simulink model "DFADAS2_SenFus_v1_201204RC_training_210115"  (R2018b)
settings: Solver=FixedStepDiscrete  StartTime=0.0  StopTime=inf  FixedStep=0.002  RelTol=1e-3  EnableMultiTasking=on
PreLoadFcn:
  | RTWConfigurationCB('preloadfcn', bdroot);
libraries: canmsglib x108, simulink x48, canfdmsglib x12
(part 12 of 28)

== system DFADAS2_SenFus_v1_201204RC_training_210115/Signal Input (Input)/Signal Input (10ms) (Input10)/VehInfo/Vehicle Movement Signal Receive and Processing (VehMovRx)/Yaw State CAN Frame PreProcess (YawCANFrmPPrcs) ==
  CAN Diagnosis (CANDia) : Subsystem  Commented=on
  CAN Receive Sample Time : Constant  Value=0.02  OutDataTypeStr=single  SampleTime=-1
  CAN Unpack : canmsglib/CAN Unpack  CANdbFile=F:\LD\3_simulinkModel_13b\TJAHWA\ADAS_D53_PSA1CAN_LiPiao_DLC.dbc  MsgList=ESC_3CD_PSA1  MsgName=ESC_3CD_PSA1  MsgIDType=Standard (11-bit identifier)  MsgIdentifier=973  MsgLength=8  SignalInfo=Brake_pedal_disabled_UC_Brake$37$1$2$2$1$0$1$0$-Inf$Inf$#Frame_checksum3CD$60$4$2$2$1$0$1$0$-Inf$Inf$#Lateral_acceleration$8$16$2$1$1$0$5.000000e-02$0$-15$15$#TMC_pressure$52$12$2$2$1$0$1.000000e-01$-55$-55$3.544000e+02$#Yaw_speed$24$16$2$1$1$0$1.000000e-01$0$-100$100$#bits_compute_process_counter3CD$56$4$2$2$1$0$1$0$0$15$#  NSignals=6  IDPort=off  TimestampPort=off  ErrorPort=off  RemotePort=off  LengthPort=off  StatusPort=off  StartBits=str2num('[int32(37);int32(60);int32(8);int32(52);int32(24);int32(56)]')  SignalSizes=str2num('[int32(1);int32(4);int32(16);int32(12);int32(16);int32(4)]')  ByteOrders=str2num('[int32(2);int32(2);int32(2);int32(2);int32(2);int32(2)]')  DataTypes=str2num('[int32(2);int32(2);int32(1);int32(2);int32(1);int32(2)]')  MultiplexTypes=str2num('[int32(1);int32(1);int32(1);int32(1);int32(1);int32(1)]')  MultiplexValues=str2num('[double(0);double(0);double(0);double(0);double(0);double(0)]')  Factors=str2num('[double(1);double(1);double(5.000000e-02);double(1.000000e-01);double(1.000000e-01);double(1)]')  Offsets=str2num('[double(0);double(0);double(0);double(-55);double(0);double(0)]')  Minimums=str2num('[double(-Inf);double(-Inf);double(-15);double(-55);double(-100);double(0)]')  Maximums=str2num('[double(Inf);double(Inf);double(15);double(3.544000e+02);double(100);double(15)]')  ApplyMinMax=off
      settings: SourceProductName=Simulink Real-Time  SourceProductBaseCode=XP  DataFormat=CANdb specified signals
  Data Type Conversion{2..5} (4 alike) : DataTypeConversion  OutDataTypeStr=single
  Data Type Conversion55 : DataTypeConversion  OutDataTypeStr=uint16
  Rate Transition{1..5} (5 alike) : RateTransition  OutPortSampleTime=0.01
  S-Function1 : S-Function  FunctionName=NSTC297CANReceiveBlkLib  Parameters=|  SFunctionDeploymentMode=off  EnableBusSupport=off  mask(NSTC297 CAN Receive){Ns_DeviceID=ADAS Control Unit Gen2, Ns_ChannelNum=4, Ns_FrameID=973, Ns_IsVirtualFrame=off, Ns_RoleInVirtualFrame=Header Frame, Ns_HeaderFrameID=0, Ns_VirtualFrameStatusFlg=off, Ns_IncompleteFrameCntFlg=off, Ns_OverflowCntFlg=off, Ns_FrameBufferSize=1, Ns_SampleTime=0.01}
      | uint16(Ns_DeviceID),
      | uint16(Ns_ChannelNum),
      | uint32(Ns_FrameID),
      | uint8(Ns_IsVirtualFrame),
      | uint16(Ns_RoleInVirtualFrame),
      | uint32(Ns_HeaderFrameID),
      | uint8(Ns_VirtualFrameStatusFlg),
      | uint8(Ns_IncompleteFrameCntFlg),
      | uint8(Ns_OverflowCntFlg),
      | uint16(Ns_FrameBufferSize),
      | double(Ns_SampleTime)
      mask prompts: Ns_DeviceID "Device:"; Ns_ChannelNum "Channel number:"; Ns_FrameID "Frame ID:"; Ns_IsVirtualFrame "Belong to a virtual frame"; Ns_RoleInVirtualFrame "Position in virtual frame:"; Ns_HeaderFrameID "Header frame ID:"; Ns_VirtualFrameStatusFlg "Current virtural frame status output"; Ns_IncompleteFrameCntFlg "Incomplete virtual frame count output"; Ns_OverflowCntFlg "Overflow count output"; Ns_FrameBufferSize "Frame buffer size:"; Ns_SampleTime "Sample time:"
      mask init:
      | NSTC297CANReceive_callback('portlabels');
      mask TypeOptions Ns_DeviceID: General Control Unit Gen2 | ADAS Control Unit Gen2
      mask TypeOptions Ns_ChannelNum: 0 | 1 | 2 | 3 | 4 | 5
      mask Callback Ns_IsVirtualFrame: NSTC297CANReceive_callback('Belong to a virtual frame');
      mask TypeOptions Ns_RoleInVirtualFrame: Header Frame | Data Frame | Trailer Frame
      mask Callback Ns_RoleInVirtualFrame: NSTC297CANReceive_callback('Position in virtual frame');
      mask Display: color('blue');text(0.02,0.9,'NovSteeds TC297','horizontalAlignment','left');color('blue');text(0.5,0.7,'CAN Receive','horizontalAlignment','center');color('black');text(0.5,0.6,'Channel: 4','horizontalAlignment','center');text(0.5,0.5,'ID: 973','horizontalAlignment','center');text(0.5,0.4,'Virtual Frame: No','horizontalAlignment','center');port_label('output',1, 'RemainderCnt');port_label('output',2, 'Msg');
  Time Limit : Constant  OutDataTypeStr=single  SampleTime=-1
  YawCANFrmPPrcs_aLAcc : Outport
  Brake_pedal_disabled_UC_Brake : Outport  Port=2
  YawCANFrmPPrcs_arYR : Outport  Port=3
  Out4 : Outport  Port=4
  Out5 : Outport  Port=5
  wires:
  CAN Receive Sample Time/1 -> CAN Diagnosis (CANDia)/1(CANDia_tiCANRxSmplT)
  Time Limit/1 -> CAN Diagnosis (CANDia)/2(CANDia_tiTLim)
  S-Function1/1 -> CAN Diagnosis (CANDia)/3(CANDia_cfNewFlg)
  S-Function1/2 -> CAN Unpack/1, CAN Diagnosis (CANDia)/4(CANDia_regCANMsg)
  Rate Transition3/1 -> Data Type Conversion3/1
  Data Type Conversion3/1 -> YawCANFrmPPrcs_aLAcc/1
  Rate Transition1/1 -> Data Type Conversion55/1
  Rate Transition2/1 -> Data Type Conversion2/1
  Rate Transition4/1 -> Data Type Conversion4/1
  Rate Transition5/1 -> Data Type Conversion5/1
  Data Type Conversion2/1 -> YawCANFrmPPrcs_arYR/1
  Data Type Conversion4/1 -> Out4/1
  Data Type Conversion5/1 -> Out5/1
  CAN Unpack/3 -> Rate Transition3/1
  CAN Unpack/5 -> Rate Transition2/1
  Data Type Conversion55/1 -> Brake_pedal_disabled_UC_Brake/1
  CAN Unpack/1 -> Rate Transition1/1

== system DFADAS2_SenFus_v1_201204RC_training_210115/Signal Input (Input)/Signal Input (50ms) (Input50)/Cmr/CmrInfo/L0 Information (L0Info)  ==
  CAN Diagnosis (CANDia)1 : Subsystem  Commented=on
  CAN Receive (CANRX)2 : S-Function  Commented=on  FunctionName=CAN_Rec_P  Parameters=uint8(Module-1),uint32(ID),uint8(Frameformat-1),uint8(Newflag),uint8(FIFO),double(sampletime)  SFunctionDeploymentMode=off  EnableBusSupport=off  mask(CAN_receive){Module=CAN_2, ID=1530, Frameformat=Extended (29-bit identifier), Newflag=on, FIFO=off, sampletime=0.01}
      mask prompts: Module "CAN Port:"; ID "CAN Frame ID:"; Frameformat "CAN Frame Format:"; FIFO "Overflow flag"
      mask init:
      | maskdisplay = canrecicon(Module,ID,Frameformat,Newflag,FIFO);
      | set_param(gcb, 'MaskDisplay', maskdisplay);
      mask TypeOptions Module: CAN_0 | CAN_1 | CAN_2 | CAN_3
      mask TypeOptions Frameformat: Standard (11-bit identifier) | Extended (29-bit identifier)
      mask Display: color('blue');text(0.98,0.9,'MPC5675K','horizontalAlignment','right');color('black');text(0.5,0.6,'FlexCAN_2 Receive','horizontalAlignment','center');text(0.5,0.35,'Extended ID:1530','horizontalAlignment','center');port_label('output',1,'New_Flag');port_label('output',2,'CAN_Msg');
  CAN Receive (CANRX)3 : S-Function  Commented=on  FunctionName=CAN_Rec_P  Parameters=uint8(Module-1),uint32(ID),uint8(Frameformat-1),uint8(Newflag),uint8(FIFO),double(sampletime)  SFunctionDeploymentMode=off  EnableBusSupport=off  mask(CAN_receive){Module=CAN_2, ID=1532, Frameformat=Extended (29-bit identifier), Newflag=on, FIFO=off, sampletime=0.01}
      mask prompts: Module "CAN Port:"; ID "CAN Frame ID:"; Frameformat "CAN Frame Format:"; FIFO "Overflow flag"
      mask init:
      | maskdisplay = canrecicon(Module,ID,Frameformat,Newflag,FIFO);
      | set_param(gcb, 'MaskDisplay', maskdisplay);
      mask TypeOptions Module: CAN_0 | CAN_1 | CAN_2 | CAN_3
      mask TypeOptions Frameformat: Standard (11-bit identifier) | Extended (29-bit identifier)
      mask Display: color('blue');text(0.98,0.9,'MPC5675K','horizontalAlignment','right');color('black');text(0.5,0.6,'FlexCAN_2 Receive','horizontalAlignment','center');text(0.5,0.35,'Extended ID:1532','horizontalAlignment','center');port_label('output',1,'New_Flag');port_label('output',2,'CAN_Msg');
  CAN Receive Sample Time1 : Constant  Commented=on  Value=0.02  OutDataTypeStr=single  SampleTime=-1
  CAN Unpack2 : canmsglib/CAN Unpack  Commented=on  CANdbFile=F:\LD\1_simulinkModel_10b\LKA\LKA_All\Video_Fusion.dbc  MsgList=Video_Lane_Left_B  MsgName=Video_Lane_Left_B  MsgIDType=Standard (11-bit identifier)  MsgIdentifier=1532  MsgLength=4  SignalInfo=Line_Width$17$7$2$2$1$0$1.000000e-02$0$0$1.270000e+00$#Me_Line_Changed$16$1$2$2$1$0$1$0$0$1$#Message_Counter$30$2$2$2$1$0$1$0$0$3$#TLC$8$8$2$2$1$0$1.000000e-02$0$0$2.550000e+00$#View_Range$0$8$2$2$1$0$5.000000e-01$0$0$1.275000e+02$#  NSignals=5  IDPort=off  TimestampPort=off  ErrorPort=off  RemotePort=off  LengthPort=off  StatusPort=off  StartBits=str2num('[int32(17);int32(16);int32(30);int32(8);int32(0)]')  SignalSizes=str2num('[int32(7);int32(1);int32(2);int32(8);int32(8)]')  ByteOrders=str2num('[int32(2);int32(2);int32(2);int32(2);int32(2)]')  DataTypes=str2num('[int32(2);int32(2);int32(2);int32(2);int32(2)]')  MultiplexTypes=str2num('[int32(1);int32(1);int32(1);int32(1);int32(1)]')  MultiplexValues=str2num('[double(0);double(0);double(0);double(0);double(0)]')  Factors=str2num('[double(1.000000e-02);double(1);double(1);double(1.000000e-02);double(5.000000e-01)]')  Offsets=str2num('[double(0);double(0);double(0);double(0);double(0)]')  Minimums=str2num('[double(0);double(0);double(0);double(0);double(0)]')  Maximums=str2num('[double(1.270000e+00);double(1);double(3);double(2.550000e+00);double(1.275000e+02)]')  ApplyMinMax=off
      settings: SourceProductName=Simulink Real-Time  SourceProductBaseCode=XP  DataFormat=CANdb specified signals
  CAN Unpack3 : canmsglib/CAN Unpack  Commented=on  CANdbFile=F:\LD\3_simulinkModel_13b\TJAHWA\ADAS_D53_S_CAN_V2_v20190314.dbc  MsgList=Video_Lane_Left_A  MsgName=Video_Lane_Left_A  MsgIDType=Standard (11-bit identifier)  MsgIdentifier=1530  MsgLength=8  SignalInfo=C0_5FA$44$12$2$1$1$0$1.000000e-02$0$-2.048000e+01$2.047000e+01$#C1_5FA$50$10$2$1$1$0$9.765625e-04$0$-3.570000e-01$3.570000e-01$#C2_5FA$24$16$2$1$1$0$1.000000e-06$0$-3.276800e-02$3.276600e-02$#C3_5FA$8$16$2$1$1$0$4.000000e-09$0$-1.310720e-04$1.310680e-04$#Line_Type_5FA$59$3$2$2$1$0$1$0$0$7$#Message_Counter_5FA$48$2$2$2$1$0$1$0$0$3$#Quality_5FA$62$2$2$2$1$0$1$0$0$3$#  NSignals=7  IDPort=off  TimestampPort=off  ErrorPort=off  RemotePort=off  LengthPort=off  StatusPort=off  StartBits=str2num('[int32(44);int32(50);int32(24);int32(8);int32(59);int32(48);int32(62)]')  SignalSizes=str2num('[int32(12);int32(10);int32(16);int32(16);int32(3);int32(2);int32(2)]')  ByteOrders=str2num('[int32(2);int32(2);int32(2);int32(2);int32(2);int32(2);int32(2)]')  DataTypes=str2num('[int32(1);int32(1);int32(1);int32(1);int32(2);int32(2);int32(2)]')  MultiplexTypes=str2num('[int32(1);int32(1);int32(1);int32(1);int32(1);int32(1);int32(1)]')  MultiplexValues=str2num('[double(0);double(0);double(0);double(0);double(0);double(0);double(0)]')  Factors=str2num('[double(1.000000e-02);double(9.765625e-04);double(1.000000e-06);double(4.000000e-09);double(1);double(1);double(1)]')  Offsets=str2num('[double(0);double(0);double(0);double(0);double(0);double(0);double(0)]')  Minimums=str2num('[double(-2.048000e+01);double(-3.570000e-01);double(-3.276800e-02);double(-1.310720e-04);double(0);double(0);double(0)]')  Maximums=str2num('[double(2.047000e+01);double(3.570000e-01);double(3.276600e-02);double(1.310680e-04);double(7);double(3);double(3)]')  ApplyMinMax=off
      settings: SourceProductName=Simulink Real-Time  SourceProductBaseCode=XP  DataFormat=CANdb specified signals
  CAN Unpack7 : canmsglib/CAN Unpack  CANdbFile=F:\V_control\ADAS ECU-Sensor CAN_V2_20190314(1).dbc  MsgList=Video_Lane_Left_A  MsgName=Video_Lane_Left_A  MsgIDType=Standard (11-bit identifier)  MsgIdentifier=1530  MsgLength=8  SignalInfo=C0_5FA$44$12$2$1$1$0$1.000000e-02$0$-2.048000e+01$2.047000e+01$#C1_5FA$50$10$2$1$1$0$9.765625e-04$0$-3.570000e-01$3.570000e-01$#C2_5FA$24$16$2$1$1$0$1.000000e-06$0$-3.276800e-02$3.276600e-02$#C3_5FA$8$16$2$1$1$0$4.000000e-09$0$-1.310720e-04$1.310680e-04$#Line_Type_5FA$59$3$2$2$1$0$1$0$0$7$#Message_Counter_5FA$48$2$2$2$1$0$1$0$0$3$#Quality_5FA$62$2$2$2$1$0$1$0$0$3$#  NSignals=7  IDPort=off  TimestampPort=off  ErrorPort=off  RemotePort=off  LengthPort=off  StatusPort=off  StartBits=str2num('[int32(44);int32(50);int32(24);int32(8);int32(59);int32(48);int32(62)]')  SignalSizes=str2num('[int32(12);int32(10);int32(16);int32(16);int32(3);int32(2);int32(2)]')  ByteOrders=str2num('[int32(2);int32(2);int32(2);int32(2);int32(2);int32(2);int32(2)]')  DataTypes=str2num('[int32(1);int32(1);int32(1);int32(1);int32(2);int32(2);int32(2)]')  MultiplexTypes=str2num('[int32(1);int32(1);int32(1);int32(1);int32(1);int32(1);int32(1)]')  MultiplexValues=str2num('[double(0);double(0);double(0);double(0);double(0);double(0);double(0)]')  Factors=str2num('[double(1.000000e-02);double(9.765625e-04);double(1.000000e-06);double(4.000000e-09);double(1);double(1);double(1)]')  Offsets=str2num('[double(0);double(0);double(0);double(0);double(0);double(0);double(0)]')  Minimums=str2num('[double(-2.048000e+01);double(-3.570000e-01);double(-3.276800e-02);double(-1.310720e-04);double(0);double(0);double(0)]')  Maximums=str2num('[double(2.047000e+01);double(3.570000e-01);double(3.276600e-02);double(1.310680e-04);double(7);double(3);double(3)]')  ApplyMinMax=off
      settings: SourceProductName=Simulink Real-Time  SourceProductBaseCode=XP  DataFormat=CANdb specified signals
  Constant : Constant
  Data Type Conversion{,1..3,5} (5 alike) : DataTypeConversion  OutDataTypeStr=single
  Data Type Conversion4 : DataTypeConversion  OutDataTypeStr=uint16
  L0 Information Fault Synthesis (L0FaultSyn)1 : Subsystem
  S-Function6 : S-Function  FunctionName=NSTC297CANReceiveBlkLib  Parameters=|  SFunctionDeploymentMode=off  EnableBusSupport=off  mask(NSTC297 CAN Receive){Ns_DeviceID=ADAS Control Unit Gen2, Ns_ChannelNum=5, Ns_FrameID=1530, Ns_IsVirtualFrame=off, Ns_RoleInVirtualFrame=Header Frame, Ns_HeaderFrameID=0, Ns_VirtualFrameStatusFlg=off, Ns_IncompleteFrameCntFlg=off, Ns_OverflowCntFlg=off, Ns_FrameBufferSize=1, Ns_SampleTime=0.05}
      | uint16(Ns_DeviceID),
      | uint16(Ns_ChannelNum),
      | uint32(Ns_FrameID),
      | uint8(Ns_IsVirtualFrame),
      | uint16(Ns_RoleInVirtualFrame),
      | uint32(Ns_HeaderFrameID),
      | uint8(Ns_VirtualFrameStatusFlg),
      | uint8(Ns_IncompleteFrameCntFlg),
      | uint8(Ns_OverflowCntFlg),
      | uint16(Ns_FrameBufferSize),
      | double(Ns_SampleTime)
      mask prompts: Ns_DeviceID "Device:"; Ns_ChannelNum "Channel number:"; Ns_FrameID "Frame ID:"; Ns_IsVirtualFrame "Belong to a virtual frame"; Ns_RoleInVirtualFrame "Position in virtual frame:"; Ns_HeaderFrameID "Header frame ID:"; Ns_VirtualFrameStatusFlg "Current virtural frame status output"; Ns_IncompleteFrameCntFlg "Incomplete virtual frame count output"; Ns_OverflowCntFlg "Overflow count output"; Ns_FrameBufferSize "Frame buffer size:"; Ns_SampleTime "Sample time:"
      mask init:
      | NSTC297CANReceive_callback('portlabels');
      mask TypeOptions Ns_DeviceID: General Control Unit Gen2 | ADAS Control Unit Gen2
      mask TypeOptions Ns_ChannelNum: 0 | 1 | 2 | 3 | 4 | 5
      mask Callback Ns_IsVirtualFrame: NSTC297CANReceive_callback('Belong to a virtual frame');
      mask TypeOptions Ns_RoleInVirtualFrame: Header Frame | Data Frame | Trailer Frame
      mask Callback Ns_RoleInVirtualFrame: NSTC297CANReceive_callback('Position in virtual frame');
      mask Display: color('blue');text(0.02,0.9,'NovSteeds TC297','horizontalAlignment','left');color('blue');text(0.5,0.7,'CAN Receive','horizontalAlignment','center');color('black');text(0.5,0.6,'Channel: 5','horizontalAlignment','center');text(0.5,0.5,'ID: 1530','horizontalAlignment','center');text(0.5,0.4,'Virtual Frame: No','horizontalAlignment','center');port_label('output',1, 'RemainderCnt');port_label('output',2, 'Msg');
  Time Limit1 : Constant  Commented=on  OutDataTypeStr=single  SampleTime=-1
  L0Info_facmL0C0 : Outport
  L0Info_facmL0C1 : Outport  Port=2
  L0Info_facmL0C2 : Outport  Port=3
  L0Info_facmL0C3 : Outport  Port=4
  L0Info_facmL0Ql : Outport  Port=5
  L0Info_facmL0Rng : Outport  Port=6
  L0Info_efL0FaultSyn : Outport  Port=7
  wires:
  Data Type Conversion1/1 -> L0Info_facmL0C1/1
  Data Type Conversion2/1 -> L0Info_facmL0C2/1
  Data Type Conversion3/1 -> L0Info_facmL0C3/1
  Data Type Conversion4/1 -> L0Info_facmL0Ql/1
  Data Type Conversion/1 -> L0Info_facmL0C0/1
  Data Type Conversion5/1 -> L0Info_facmL0Rng/1
  CAN Receive (CANRX)3/2 -> CAN Unpack2/1
  ? -> CAN Diagnosis (CANDia)1/5(CANDia_ctRllCnt)
  CAN Receive Sample Time1/1 -> CAN Diagnosis (CANDia)1/1(CANDia_tiCANRxSmplT)
  Time Limit1/1 -> CAN Diagnosis (CANDia)1/2(CANDia_tiTLim)
  CAN Receive (CANRX)2/1 -> CAN Diagnosis (CANDia)1/3(CANDia_cfNewFlg)
  CAN Receive (CANRX)2/2 -> CAN Diagnosis (CANDia)1/4(CANDia_regCANMsg), CAN Unpack3/1
  CAN Unpack7/2 -> Data Type Conversion1/1
  CAN Unpack7/3 -> Data Type Conversion2/1
  CAN Unpack7/4 -> Data Type Conversion3/1
  CAN Unpack7/1 -> Data Type Conversion/1
  CAN Unpack7/7 -> Data Type Conversion4/1
  S-Function6/2 -> CAN Unpack7/1
  Constant/1 -> Data Type Conversion5/1
  L0 Information Fault Synthesis (L0FaultSyn)1/1(L0FaultSyn_efL0FaultSyn) -> L0Info_efL0FaultSyn/1

== system DFADAS2_SenFus_v1_201204RC_training_210115/Signal Input (Input)/Signal Input (50ms) (Input50)/Cmr/CmrInfo/L1 Information (L1Info) ==
  CAN Diagnosis (CANDia) : Subsystem  Commented=on
  CAN Receive (CANRX) : S-Function  Commented=on  FunctionName=CAN_Rec_P  Parameters=uint8(Module-1),uint32(ID),uint8(Frameformat-1),uint8(Newflag),uint8(FIFO),double(sampletime)  SFunctionDeploymentMode=off  EnableBusSupport=off  mask(CAN_receive){Module=CAN_2, ID=1531, Frameformat=Extended (29-bit identifier), Newflag=on, FIFO=off, sampletime=0.01}
      mask prompts: Module "CAN Port:"; ID "CAN Frame ID:"; Frameformat "CAN Frame Format:"; FIFO "Overflow flag"
      mask init:
      | maskdisplay = canrecicon(Module,ID,Frameformat,Newflag,FIFO);
      | set_param(gcb, 'MaskDisplay', maskdisplay);
      mask TypeOptions Module: CAN_0 | CAN_1 | CAN_2 | CAN_3
      mask TypeOptions Frameformat: Standard (11-bit identifier) | Extended (29-bit identifier)
      mask Display: color('blue');text(0.98,0.9,'MPC5675K','horizontalAlignment','right');color('black');text(0.5,0.6,'FlexCAN_2 Receive','horizontalAlignment','center');text(0.5,0.35,'Extended ID:1531','horizontalAlignment','center');port_label('output',1,'New_Flag');port_label('output',2,'CAN_Msg');
  CAN Receive Sample Time : Constant  Commented=on  Value=0.02  OutDataTypeStr=single  SampleTime=-1
  CAN Unpack1 : canmsglib/CAN Unpack  CANdbFile=F:\V_control\ADAS ECU-Sensor CAN_V2_20190314(1).dbc  MsgList=Video_Lane_Next_Left_A  MsgName=Video_Lane_Next_Left_A  MsgIDType=Standard (11-bit identifier)  MsgIdentifier=1531  MsgLength=8  SignalInfo=C0_5FB$44$12$2$1$1$0$1.000000e-02$0$-2.048000e+01$2.047000e+01$#C1_5FB$50$10$2$1$1$0$9.765625e-04$0$-3.570000e-01$3.570000e-01$#C2_5FB$24$16$2$1$1$0$1.000000e-06$0$-3.276800e-02$3.276600e-02$#C3_5FB$8$16$2$1$1$0$4.000000e-09$0$-1.310720e-04$1.310680e-04$#Line_Type_5FB$59$3$2$2$1$0$1$0$0$7$#Message_Counter_5FB$48$2$2$2$1$0$1$0$0$3$#Quality_5FB$62$2$2$2$1$0$1$0$0$3$#  NSignals=7  IDPort=off  TimestampPort=off  ErrorPort=off  RemotePort=off  LengthPort=off  StatusPort=off  StartBits=str2num('[int32(44);int32(50);int32(24);int32(8);int32(59);int32(48);int32(62)]')  SignalSizes=str2num('[int32(12);int32(10);int32(16);int32(16);int32(3);int32(2);int32(2)]')  ByteOrders=str2num('[int32(2);int32(2);int32(2);int32(2);int32(2);int32(2);int32(2)]')  DataTypes=str2num('[int32(1);int32(1);int32(1);int32(1);int32(2);int32(2);int32(2)]')  MultiplexTypes=str2num('[int32(1);int32(1);int32(1);int32(1);int32(1);int32(1);int32(1)]')  MultiplexValues=str2num('[double(0);double(0);double(0);double(0);double(0);double(0);double(0)]')  Factors=str2num('[double(1.000000e-02);double(9.765625e-04);double(1.000000e-06);double(4.000000e-09);double(1);double(1);double(1)]')  Offsets=str2num('[double(0);double(0);double(0);double(0);double(0);double(0);double(0)]')  Minimums=str2num('[double(-2.048000e+01);double(-3.570000e-01);double(-3.276800e-02);double(-1.310720e-04);double(0);double(0);double(0)]')  Maximums=str2num('[double(2.047000e+01);double(3.570000e-01);double(3.276600e-02);double(1.310680e-04);double(7);double(3);double(3)]')  ApplyMinMax=off
      settings: SourceProductName=Simulink Real-Time  SourceProductBaseCode=XP  DataFormat=CANdb specified signals
  CAN Unpack13 : canmsglib/CAN Unpack  Commented=on  CANdbFile=F:\LD\3_simulinkModel_13b\TJAHWA\ADAS_D53_S_CAN_V2_v20190314.dbc  MsgList=Video_Lane_Next_Left_A  MsgName=Video_Lane_Next_Left_A  MsgIDType=Standard (11-bit identifier)  MsgIdentifier=1531  MsgLength=8  SignalInfo=C0_5FB$44$12$2$1$1$0$1.000000e-02$0$-2.048000e+01$2.047000e+01$#C1_5FB$50$10$2$1$1$0$9.765625e-04$0$-3.570000e-01$3.570000e-01$#C2_5FB$24$16$2$1$1$0$1.000000e-06$0$-3.276800e-02$3.276600e-02$#C3_5FB$8$16$2$1$1$0$4.000000e-09$0$-1.310720e-04$1.310680e-04$#Line_Type_5FB$59$3$2$2$1$0$1$0$0$7$#Message_Counter_5FB$48$2$2$2$1$0$1$0$0$3$#Quality_5FB$62$2$2$2$1$0$1$0$0$3$#  NSignals=7  IDPort=off  TimestampPort=off  ErrorPort=off  RemotePort=off  LengthPort=off  StatusPort=off  StartBits=str2num('[int32(44);int32(50);int32(24);int32(8);int32(59);int32(48);int32(62)]')  SignalSizes=str2num('[int32(12);int32(10);int32(16);int32(16);int32(3);int32(2);int32(2)]')  ByteOrders=str2num('[int32(2);int32(2);int32(2);int32(2);int32(2);int32(2);int32(2)]')  DataTypes=str2num('[int32(1);int32(1);int32(1);int32(1);int32(2);int32(2);int32(2)]')  MultiplexTypes=str2num('[int32(1);int32(1);int32(1);int32(1);int32(1);int32(1);int32(1)]')  MultiplexValues=str2num('[double(0);double(0);double(0);double(0);double(0);double(0);double(0)]')  Factors=str2num('[double(1.000000e-02);double(9.765625e-04);double(1.000000e-06);double(4.000000e-09);double(1);double(1);double(1)]')  Offsets=str2num('[double(0);double(0);double(0);double(0);double(0);double(0);double(0)]')  Minimums=str2num('[double(-2.048000e+01);double(-3.570000e-01);double(-3.276800e-02);double(-1.310720e-04);double(0);double(0);double(0)]')  Maximums=str2num('[double(2.047000e+01);double(3.570000e-01);double(3.276600e-02);double(1.310680e-04);double(7);double(3);double(3)]')  ApplyMinMax=off
      settings: SourceProductName=Simulink Real-Time  SourceProductBaseCode=XP  DataFormat=CANdb specified signals
  Data Type Conversion{,1..3} (4 alike) : DataTypeConversion  OutDataTypeStr=single
  Data Type Conversion4 : DataTypeConversion  OutDataTypeStr=uint16
  L0 Information Fault Synthesis (L0FaultSyn) : Subsystem
  S-Function1 : S-Function  FunctionName=NSTC297CANReceiveBlkLib  Parameters=|  SFunctionDeploymentMode=off  EnableBusSupport=off  mask(NSTC297 CAN Receive){Ns_DeviceID=ADAS Control Unit Gen2, Ns_ChannelNum=5, Ns_FrameID=1531, Ns_IsVirtualFrame=off, Ns_RoleInVirtualFrame=Header Frame, Ns_HeaderFrameID=0, Ns_VirtualFrameStatusFlg=off, Ns_IncompleteFrameCntFlg=off, Ns_OverflowCntFlg=off, Ns_FrameBufferSize=1, Ns_SampleTime=0.05}
      | uint16(Ns_DeviceID),
      | uint16(Ns_ChannelNum),
      | uint32(Ns_FrameID),
      | uint8(Ns_IsVirtualFrame),
      | uint16(Ns_RoleInVirtualFrame),
      | uint32(Ns_HeaderFrameID),
      | uint8(Ns_VirtualFrameStatusFlg),
      | uint8(Ns_IncompleteFrameCntFlg),
      | uint8(Ns_OverflowCntFlg),
      | uint16(Ns_FrameBufferSize),
      | double(Ns_SampleTime)
      mask prompts: Ns_DeviceID "Device:"; Ns_ChannelNum "Channel number:"; Ns_FrameID "Frame ID:"; Ns_IsVirtualFrame "Belong to a virtual frame"; Ns_RoleInVirtualFrame "Position in virtual frame:"; Ns_HeaderFrameID "Header frame ID:"; Ns_VirtualFrameStatusFlg "Current virtural frame status output"; Ns_IncompleteFrameCntFlg "Incomplete virtual frame count output"; Ns_OverflowCntFlg "Overflow count output"; Ns_FrameBufferSize "Frame buffer size:"; Ns_SampleTime "Sample time:"
      mask init:
      | NSTC297CANReceive_callback('portlabels');
      mask TypeOptions Ns_DeviceID: General Control Unit Gen2 | ADAS Control Unit Gen2
      mask TypeOptions Ns_ChannelNum: 0 | 1 | 2 | 3 | 4 | 5
      mask Callback Ns_IsVirtualFrame: NSTC297CANReceive_callback('Belong to a virtual frame');
      mask TypeOptions Ns_RoleInVirtualFrame: Header Frame | Data Frame | Trailer Frame
      mask Callback Ns_RoleInVirtualFrame: NSTC297CANReceive_callback('Position in virtual frame');
      mask Display: color('blue');text(0.02,0.9,'NovSteeds TC297','horizontalAlignment','left');color('blue');text(0.5,0.7,'CAN Receive','horizontalAlignment','center');color('black');text(0.5,0.6,'Channel: 5','horizontalAlignment','center');text(0.5,0.5,'ID: 1531','horizontalAlignment','center');text(0.5,0.4,'Virtual Frame: No','horizontalAlignment','center');port_label('output',1, 'RemainderCnt');port_label('output',2, 'Msg');
  Time Limit : Constant  Commented=on  OutDataTypeStr=single  SampleTime=-1
  L1Info_facmL1C0 : Outport
  L1Info_facmL1C1 : Outport  Port=2
  L1Info_facmL1C2 : Outport  Port=3
  L1Info_facmL1C3 : Outport  Port=4
  L1Info_facmL1Ql : Outport  Port=5
  L1Info_efL1FaultSyn : Outport  Port=6
  wires:
  Data Type Conversion4/1 -> L1Info_facmL1Ql/1
  Data Type Conversion3/1 -> L1Info_facmL1C3/1
  Data Type Conversion2/1 -> L1Info_facmL1C2/1
  Data Type Conversion1/1 -> L1Info_facmL1C1/1
  ? -> CAN Diagnosis (CANDia)/5(CANDia_ctRllCnt)
  CAN Receive Sample Time/1 -> CAN Diagnosis (CANDia)/1(CANDia_tiCANRxSmplT)
  Time Limit/1 -> CAN Diagnosis (CANDia)/2(CANDia_tiTLim)
  CAN Receive (CANRX)/1 -> CAN Diagnosis (CANDia)/3(CANDia_cfNewFlg)
  CAN Receive (CANRX)/2 -> CAN Diagnosis (CANDia)/4(CANDia_regCANMsg), CAN Unpack13/1
  L0 Information Fault Synthesis (L0FaultSyn)/1(L0FaultSyn_efL0FaultSyn) -> L1Info_efL1FaultSyn/1
  Data Type Conversion/1 -> L1Info_facmL1C0/1
  S-Function1/2 -> CAN Unpack1/1
  CAN Unpack1/1 -> Data Type Conversion/1
  CAN Unpack1/2 -> Data Type Conversion1/1
  CAN Unpack1/3 -> Data Type Conversion2/1
  CAN Unpack1/4 -> Data Type Conversion3/1
  CAN Unpack1/7 -> Data Type Conversion4/1

== system DFADAS2_SenFus_v1_201204RC_training_210115/Signal Input (Input)/Signal Input (50ms) (Input50)/Cmr/CmrInfo/R0 Information (R0Info) ==
  CAN Diagnosis (CANDia) : Subsystem  Commented=on
  CAN Receive (CANRX) : S-Function  Commented=on  FunctionName=CAN_Rec_P  Parameters=uint8(Module-1),uint32(ID),uint8(Frameformat-1),uint8(Newflag),uint8(FIFO),double(sampletime)  SFunctionDeploymentMode=off  EnableBusSupport=off  mask(CAN_receive){Module=CAN_2, ID=1533, Frameformat=Extended (29-bit identifier), Newflag=on, FIFO=off, sampletime=0.01}
      mask prompts: Module "CAN Port:"; ID "CAN Frame ID:"; Frameformat "CAN Frame Format:"; FIFO "Overflow flag"
      mask init:
      | maskdisplay = canrecicon(Module,ID,Frameformat,Newflag,FIFO);
      | set_param(gcb, 'MaskDisplay', maskdisplay);
      mask TypeOptions Module: CAN_0 | CAN_1 | CAN_2 | CAN_3
      mask TypeOptions Frameformat: Standard (11-bit identifier) | Extended (29-bit identifier)
      mask Display: color('blue');text(0.98,0.9,'MPC5675K','horizontalAlignment','right');color('black');text(0.5,0.6,'FlexCAN_2 Receive','horizontalAlignment','center');text(0.5,0.35,'Extended ID:1533','horizontalAlignment','center');port_label('output',1,'New_Flag');port_label('output',2,'CAN_Msg');
  CAN Receive (CANRX)1 : S-Function  Commented=on  FunctionName=CAN_Rec_P  Parameters=uint8(Module-1),uint32(ID),uint8(Frameformat-1),uint8(Newflag),uint8(FIFO),double(sampletime)  SFunctionDeploymentMode=off  EnableBusSupport=off  mask(CAN_receive){Module=CAN_2, ID=1535, Frameformat=Extended (29-bit identifier), Newflag=on, FIFO=off, sampletime=0.01}
      mask prompts: Module "CAN Port:"; ID "CAN Frame ID:"; Frameformat "CAN Frame Format:"; FIFO "Overflow flag"
      mask init:
      | maskdisplay = canrecicon(Module,ID,Frameformat,Newflag,FIFO);
      | set_param(gcb, 'MaskDisplay', maskdisplay);
      mask TypeOptions Module: CAN_0 | CAN_1 | CAN_2 | CAN_3
      mask TypeOptions Frameformat: Standard (11-bit identifier) | Extended (29-bit identifier)
      mask Display: color('blue');text(0.98,0.9,'MPC5675K','horizontalAlignment','right');color('black');text(0.5,0.6,'FlexCAN_2 Receive','horizontalAlignment','center');text(0.5,0.35,'Extended ID:1535','horizontalAlignment','center');port_label('output',1,'New_Flag');port_label('output',2,'CAN_Msg');
  CAN Receive Sample Time : Constant  Commented=on  Value=0.02  OutDataTypeStr=single  SampleTime=-1
  CAN Unpack1 : canmsglib/CAN Unpack  Commented=on  CANdbFile=F:\LD\3_simulinkModel_13b\TJAHWA\ADAS_D53_S_CAN_V2_v20190314.dbc  MsgList=Video_Lane_Right_B  MsgName=Video_Lane_Right_B  MsgIDType=Standard (11-bit identifier)  MsgIdentifier=1535  MsgLength=4  SignalInfo=Line_Width_5FF$17$7$2$2$1$0$1.000000e-02$0$0$1.270000e+00$#Me_Line_Changed_5FF$16$1$2$2$1$0$1$0$0$1$#Message_Counter_5FF$30$2$2$2$1$0$1$0$0$3$#TLC_5FF$8$8$2$2$1$0$1.000000e-02$0$0$2.550000e+00$#View_Range_5FF$0$8$2$2$1$0$5.000000e-01$0$0$1.275000e+02$#  NSignals=5  IDPort=off  TimestampPort=off  ErrorPort=off  RemotePort=off  LengthPort=off  StatusPort=off  StartBits=str2num('[int32(17);int32(16);int32(30);int32(8);int32(0)]')  SignalSizes=str2num('[int32(7);int32(1);int32(2);int32(8);int32(8)]')  ByteOrders=str2num('[int32(2);int32(2);int32(2);int32(2);int32(2)]')  DataTypes=str2num('[int32(2);int32(2);int32(2);int32(2);int32(2)]')  MultiplexTypes=str2num('[int32(1);int32(1);int32(1);int32(1);int32(1)]')  MultiplexValues=str2num('[double(0);double(0);double(0);double(0);double(0)]')  Factors=str2num('[double(1.000000e-02);double(1);double(1);double(1.000000e-02);double(5.000000e-01)]')  Offsets=str2num('[double(0);double(0);double(0);double(0);double(0)]')  Minimums=str2num('[double(0);double(0);double(0);double(0);double(0)]')  Maximums=str2num('[double(1.270000e+00);double(1);double(3);double(2.550000e+00);double(1.275000e+02)]')  ApplyMinMax=off
      settings: SourceProductName=Simulink Real-Time  SourceProductBaseCode=XP  DataFormat=CANdb specified signals
  CAN Unpack14 : canmsglib/CAN Unpack  Commented=on  CANdbFile=F:\LD\3_simulinkModel_13b\TJAHWA\ADAS_D53_S_CAN_V2_v20190314.dbc  MsgList=Video_Lane_Right_A  MsgName=Video_Lane_Right_A  MsgIDType=Standard (11-bit identifier)  MsgIdentifier=1533  MsgLength=8  SignalInfo=C0_5FD$44$12$2$1$1$0$1.000000e-02$0$-2.048000e+01$2.047000e+01$#C1_5FD$50$10$2$1$1$0$9.765625e-04$0$-3.570000e-01$3.570000e-01$#C2_5FD$24$16$2$1$1$0$1.000000e-06$0$-3.276800e-02$3.276600e-02$#C3_5FD$8$16$2$1$1$0$4.000000e-09$0$-1.310720e-04$1.310680e-04$#Line_Type_5FD$59$3$2$2$1$0$1$0$0$7$#Message_Counter_5FD$48$2$2$2$1$0$1$0$0$3$#Quality_5FD$62$2$2$2$1$0$1$0$0$3$#  NSignals=7  IDPort=off  TimestampPort=off  ErrorPort=off  RemotePort=off  LengthPort=off  StatusPort=off  StartBits=str2num('[int32(44);int32(50);int32(24);int32(8);int32(59);int32(48);int32(62)]')  SignalSizes=str2num('[int32(12);int32(10);int32(16);int32(16);int32(3);int32(2);int32(2)]')  ByteOrders=str2num('[int32(2);int32(2);int32(2);int32(2);int32(2);int32(2);int32(2)]')  DataTypes=str2num('[int32(1);int32(1);int32(1);int32(1);int32(2);int32(2);int32(2)]')  MultiplexTypes=str2num('[int32(1);int32(1);int32(1);int32(1);int32(1);int32(1);int32(1)]')  MultiplexValues=str2num('[double(0);double(0);double(0);double(0);double(0);double(0);double(0)]')  Factors=str2num('[double(1.000000e-02);double(9.765625e-04);double(1.000000e-06);double(4.000000e-09);double(1);double(1);double(1)]')  Offsets=str2num('[double(0);double(0);double(0);double(0);double(0);double(0);double(0)]')  Minimums=str2num('[double(-2.048000e+01);double(-3.570000e-01);double(-3.276800e-02);double(-1.310720e-04);double(0);double(0);double(0)]')  Maximums=str2num('[double(2.047000e+01);double(3.570000e-01);double(3.276600e-02);double(1.310680e-04);double(7);double(3);double(3)]')  ApplyMinMax=off
      settings: SourceProductName=Simulink Real-Time  SourceProductBaseCode=XP  DataFormat=CANdb specified signals
  CAN Unpack2 : canmsglib/CAN Unpack  CANdbFile=F:\V_control\ADAS ECU-Sensor CAN_V2_20190314(1).dbc  MsgList=Video_Lane_Right_A  MsgName=Video_Lane_Right_A  MsgIDType=Standard (11-bit identifier)  MsgIdentifier=1533  MsgLength=8  SignalInfo=C0_5FD$44$12$2$1$1$0$1.000000e-02$0$-2.048000e+01$2.047000e+01$#C1_5FD$50$10$2$1$1$0$9.765625e-04$0$-3.570000e-01$3.570000e-01$#C2_5FD$24$16$2$1$1$0$1.000000e-06$0$-3.276800e-02$3.276600e-02$#C3_5FD$8$16$2$1$1$0$4.000000e-09$0$-1.310720e-04$1.310680e-04$#Line_Type_5FD$59$3$2$2$1$0$1$0$0$7$#Message_Counter_5FD$48$2$2$2$1$0$1$0$0$3$#Quality_5FD$62$2$2$2$1$0$1$0$0$3$#  NSignals=7  IDPort=off  TimestampPort=off  ErrorPort=off  RemotePort=off  LengthPort=off  StatusPort=off  StartBits=str2num('[int32(44);int32(50);int32(24);int32(8);int32(59);int32(48);int32(62)]')  SignalSizes=str2num('[int32(12);int32(10);int32(16);int32(16);int32(3);int32(2);int32(2)]')  ByteOrders=str2num('[int32(2);int32(2);int32(2);int32(2);int32(2);int32(2);int32(2)]')  DataTypes=str2num('[int32(1);int32(1);int32(1);int32(1);int32(2);int32(2);int32(2)]')  MultiplexTypes=str2num('[int32(1);int32(1);int32(1);int32(1);int32(1);int32(1);int32(1)]')  MultiplexValues=str2num('[double(0);double(0);double(0);double(0);double(0);double(0);double(0)]')  Factors=str2num('[double(1.000000e-02);double(9.765625e-04);double(1.000000e-06);double(4.000000e-09);double(1);double(1);double(1)]')  Offsets=str2num('[double(0);double(0);double(0);double(0);double(0);double(0);double(0)]')  Minimums=str2num('[double(-2.048000e+01);double(-3.570000e-01);double(-3.276800e-02);double(-1.310720e-04);double(0);double(0);double(0)]')  Maximums=str2num('[double(2.047000e+01);double(3.570000e-01);double(3.276600e-02);double(1.310680e-04);double(7);double(3);double(3)]')  ApplyMinMax=off
      settings: SourceProductName=Simulink Real-Time  SourceProductBaseCode=XP  DataFormat=CANdb specified signals
  Constant : Constant
  Data Type Conversion{1..4,6} (5 alike) : DataTypeConversion  OutDataTypeStr=single
  Data Type Conversion5 : DataTypeConversion  OutDataTypeStr=uint16
  R0 Information Fault Synthesis (R0FaultSyn) : Subsystem
  S-Function2 : S-Function  FunctionName=NSTC297CANReceiveBlkLib  Parameters=|  SFunctionDeploymentMode=off  EnableBusSupport=off  mask(NSTC297 CAN Receive){Ns_DeviceID=ADAS Control Unit Gen2, Ns_ChannelNum=5, Ns_FrameID=1533, Ns_IsVirtualFrame=off, Ns_RoleInVirtualFrame=Header Frame, Ns_HeaderFrameID=0, Ns_VirtualFrameStatusFlg=off, Ns_IncompleteFrameCntFlg=off, Ns_OverflowCntFlg=off, Ns_FrameBufferSize=1, Ns_SampleTime=0.05}
      | uint16(Ns_DeviceID),
      | uint16(Ns_ChannelNum),
      | uint32(Ns_FrameID),
      | uint8(Ns_IsVirtualFrame),
      | uint16(Ns_RoleInVirtualFrame),
      | uint32(Ns_HeaderFrameID),
      | uint8(Ns_VirtualFrameStatusFlg),
      | uint8(Ns_IncompleteFrameCntFlg),
      | uint8(Ns_OverflowCntFlg),
      | uint16(Ns_FrameBufferSize),
      | double(Ns_SampleTime)
      mask prompts: Ns_DeviceID "Device:"; Ns_ChannelNum "Channel number:"; Ns_FrameID "Frame ID:"; Ns_IsVirtualFrame "Belong to a virtual frame"; Ns_RoleInVirtualFrame "Position in virtual frame:"; Ns_HeaderFrameID "Header frame ID:"; Ns_VirtualFrameStatusFlg "Current virtural frame status output"; Ns_IncompleteFrameCntFlg "Incomplete virtual frame count output"; Ns_OverflowCntFlg "Overflow count output"; Ns_FrameBufferSize "Frame buffer size:"; Ns_SampleTime "Sample time:"
      mask init:
      | NSTC297CANReceive_callback('portlabels');
      mask TypeOptions Ns_DeviceID: General Control Unit Gen2 | ADAS Control Unit Gen2
      mask TypeOptions Ns_ChannelNum: 0 | 1 | 2 | 3 | 4 | 5
      mask Callback Ns_IsVirtualFrame: NSTC297CANReceive_callback('Belong to a virtual frame');
      mask TypeOptions Ns_RoleInVirtualFrame: Header Frame | Data Frame | Trailer Frame
      mask Callback Ns_RoleInVirtualFrame: NSTC297CANReceive_callback('Position in virtual frame');
      mask Display: color('blue');text(0.02,0.9,'NovSteeds TC297','horizontalAlignment','left');color('blue');text(0.5,0.7,'CAN Receive','horizontalAlignment','center');color('black');text(0.5,0.6,'Channel: 5','horizontalAlignment','center');text(0.5,0.5,'ID: 1533','horizontalAlignment','center');text(0.5,0.4,'Virtual Frame: No','horizontalAlignment','center');port_label('output',1, 'RemainderCnt');port_label('output',2, 'Msg');
  Time Limit : Constant  Commented=on  OutDataTypeStr=single  SampleTime=-1
  R0Info_facmR0C0 : Outport
  R0Info_facmR0C1 : Outport  Port=2
  R0Info_facmR0C2 : Outport  Port=3
  R0Info_facmR0C3 : Outport  Port=4
  R0Info_facmR0Ql : Outport  Port=5
  R0Info_facmR0Rng : Outport  Port=6
  R0Info_efR0FaultSyn : Outport  Port=7
  wires:
  R0 Information Fault Synthesis (R0FaultSyn)/1(R0FaultSyn_efL0FaultSyn) -> R0Info_efR0FaultSyn/1
  ? -> CAN Diagnosis (CANDia)/5(CANDia_ctRllCnt)
  CAN Receive Sample Time/1 -> CAN Diagnosis (CANDia)/1(CANDia_tiCANRxSmplT)
  Time Limit/1 -> CAN Diagnosis (CANDia)/2(CANDia_tiTLim)
  CAN Receive (CANRX)/1 -> CAN Diagnosis (CANDia)/3(CANDia_cfNewFlg)
  CAN Receive (CANRX)/2 -> CAN Diagnosis (CANDia)/4(CANDia_regCANMsg), CAN Unpack14/1
  Data Type Conversion1/1 -> R0Info_facmR0C1/1
  Data Type Conversion2/1 -> R0Info_facmR0C2/1
  Data Type Conversion3/1 -> R0Info_facmR0C3/1
  Data Type Conversion5/1 -> R0Info_facmR0Ql/1
  Data Type Conversion4/1 -> R0Info_facmR0C0/1
  CAN Receive (CANRX)1/2 -> CAN Unpack1/1
  Data Type Conversion6/1 -> R0Info_facmR0Rng/1
  S-Function2/2 -> CAN Unpack2/1
  CAN Unpack2/7 -> Data Type Conversion5/1
  CAN Unpack2/4 -> Data Type Conversion3/1
  CAN Unpack2/3 -> Data Type Conversion2/1
  CAN Unpack2/2 -> Data Type Conversion1/1
  CAN Unpack2/1 -> Data Type Conversion4/1
  Constant/1 -> Data Type Conversion6/1

== system DFADAS2_SenFus_v1_201204RC_training_210115/Signal Input (Input)/Signal Input (50ms) (Input50)/Cmr/CmrInfo/R1 Information (R1Info) ==
  CAN Diagnosis (CANDia) : Subsystem  Commented=on
  CAN Receive (CANRX) : S-Function  Commented=on  FunctionName=CAN_Rec_P  Parameters=uint8(Module-1),uint32(ID),uint8(Frameformat-1),uint8(Newflag),uint8(FIFO),double(sampletime)  SFunctionDeploymentMode=off  EnableBusSupport=off  mask(CAN_receive){Module=CAN_2, ID=1534, Frameformat=Extended (29-bit identifier), Newflag=on, FIFO=off, sampletime=0.01}
      mask prompts: Module "CAN Port:"; ID "CAN Frame ID:"; Frameformat "CAN Frame Format:"; FIFO "Overflow flag"
      mask init:
      | maskdisplay = canrecicon(Module,ID,Frameformat,Newflag,FIFO);
      | set_param(gcb, 'MaskDisplay', maskdisplay);
      mask TypeOptions Module: CAN_0 | CAN_1 | CAN_2 | CAN_3
      mask TypeOptions Frameformat: Standard (11-bit identifier) | Extended (29-bit identifier)
      mask Display: color('blue');text(0.98,0.9,'MPC5675K','horizontalAlignment','right');color('black');text(0.5,0.6,'FlexCAN_2 Receive','horizontalAlignment','center');text(0.5,0.35,'Extended ID:1534','horizontalAlignment','center');port_label('output',1,'New_Flag');port_label('output',2,'CAN_Msg');
  CAN Receive Sample Time : Constant  Commented=on  Value=0.02  OutDataTypeStr=single  SampleTime=-1
  CAN Unpack14 : canmsglib/CAN Unpack  Commented=on  CANdbFile=F:\LD\3_simulinkModel_13b\TJAHWA\ADAS_D53_S_CAN_V2_v20190314.dbc  MsgList=Video_Lane_Next_Right_A  MsgName=Video_Lane_Next_Right_A  MsgIDType=Standard (11-bit identifier)  MsgIdentifier=1534  MsgLength=8  SignalInfo=C0_5FE$44$12$2$1$1$0$1.000000e-02$0$-2.048000e+01$2.047000e+01$#C1_5FE$50$10$2$1$1$0$9.765625e-04$0$-3.570000e-01$3.570000e-01$#C2_5FE$24$16$2$1$1$0$1.000000e-06$0$-3.276800e-02$3.276600e-02$#C3_5FE$8$16$2$1$1$0$4.000000e-09$0$-1.310720e-04$1.310680e-04$#Line_Type_5FE$59$3$2$2$1$0$1$0$0$7$#Message_Counter_5FE$48$2$2$2$1$0$1$0$0$3$#Quality_5FE$62$2$2$2$1$0$1$0$0$3$#  NSignals=7  IDPort=off  TimestampPort=off  ErrorPort=off  RemotePort=off  LengthPort=off  StatusPort=off  StartBits=str2num('[int32(44);int32(50);int32(24);int32(8);int32(59);int32(48);int32(62)]')  SignalSizes=str2num('[int32(12);int32(10);int32(16);int32(16);int32(3);int32(2);int32(2)]')  ByteOrders=str2num('[int32(2);int32(2);int32(2);int32(2);int32(2);int32(2);int32(2)]')  DataTypes=str2num('[int32(1);int32(1);int32(1);int32(1);int32(2);int32(2);int32(2)]')  MultiplexTypes=str2num('[int32(1);int32(1);int32(1);int32(1);int32(1);int32(1);int32(1)]')  MultiplexValues=str2num('[double(0);double(0);double(0);double(0);double(0);double(0);double(0)]')  Factors=str2num('[double(1.000000e-02);double(9.765625e-04);double(1.000000e-06);double(4.000000e-09);double(1);double(1);double(1)]')  Offsets=str2num('[double(0);double(0);double(0);double(0);double(0);double(0);double(0)]')  Minimums=str2num('[double(-2.048000e+01);double(-3.570000e-01);double(-3.276800e-02);double(-1.310720e-04);double(0);double(0);double(0)]')  Maximums=str2num('[double(2.047000e+01);double(3.570000e-01);double(3.276600e-02);double(1.310680e-04);double(7);double(3);double(3)]')  ApplyMinMax=off
      settings: SourceProductName=Simulink Real-Time  SourceProductBaseCode=XP  DataFormat=CANdb specified signals
  CAN Unpack3 : canmsglib/CAN Unpack  CANdbFile=F:\V_control\ADAS ECU-Sensor CAN_V2_20190314(1).dbc  MsgList=Video_Lane_Next_Right_A  MsgName=Video_Lane_Next_Right_A  MsgIDType=Standard (11-bit identifier)  MsgIdentifier=1534  MsgLength=8  SignalInfo=C0_5FE$44$12$2$1$1$0$1.000000e-02$0$-2.048000e+01$2.047000e+01$#C1_5FE$50$10$2$1$1$0$9.765625e-04$0$-3.570000e-01$3.570000e-01$#C2_5FE$24$16$2$1$1$0$1.000000e-06$0$-3.276800e-02$3.276600e-02$#C3_5FE$8$16$2$1$1$0$4.000000e-09$0$-1.310720e-04$1.310680e-04$#Line_Type_5FE$59$3$2$2$1$0$1$0$0$7$#Message_Counter_5FE$48$2$2$2$1$0$1$0$0$3$#Quality_5FE$62$2$2$2$1$0$1$0$0$3$#  NSignals=7  IDPort=off  TimestampPort=off  ErrorPort=off  RemotePort=off  LengthPort=off  StatusPort=off  StartBits=str2num('[int32(44);int32(50);int32(24);int32(8);int32(59);int32(48);int32(62)]')  SignalSizes=str2num('[int32(12);int32(10);int32(16);int32(16);int32(3);int32(2);int32(2)]')  ByteOrders=str2num('[int32(2);int32(2);int32(2);int32(2);int32(2);int32(2);int32(2)]')  DataTypes=str2num('[int32(1);int32(1);int32(1);int32(1);int32(2);int32(2);int32(2)]')  MultiplexTypes=str2num('[int32(1);int32(1);int32(1);int32(1);int32(1);int32(1);int32(1)]')  MultiplexValues=str2num('[double(0);double(0);double(0);double(0);double(0);double(0);double(0)]')  Factors=str2num('[double(1.000000e-02);double(9.765625e-04);double(1.000000e-06);double(4.000000e-09);double(1);double(1);double(1)]')  Offsets=str2num('[double(0);double(0);double(0);double(0);double(0);double(0);double(0)]')  Minimums=str2num('[double(-2.048000e+01);double(-3.570000e-01);double(-3.276800e-02);double(-1.310720e-04);double(0);double(0);double(0)]')  Maximums=str2num('[double(2.047000e+01);double(3.570000e-01);double(3.276600e-02);double(1.310680e-04);double(7);double(3);double(3)]')  ApplyMinMax=off
      settings: SourceProductName=Simulink Real-Time  SourceProductBaseCode=XP  DataFormat=CANdb specified signals
  Data Type Conversion{1..4} (4 alike) : DataTypeConversion  OutDataTypeStr=single
  Data Type Conversion5 : DataTypeConversion  OutDataTypeStr=uint16
  R0 Information Fault Synthesis (R0FaultSyn) : Subsystem
  S-Function3 : S-Function  FunctionName=NSTC297CANReceiveBlkLib  Parameters=|  SFunctionDeploymentMode=off  EnableBusSupport=off  mask(NSTC297 CAN Receive){Ns_DeviceID=ADAS Control Unit Gen2, Ns_ChannelNum=5, Ns_FrameID=1534, Ns_IsVirtualFrame=off, Ns_RoleInVirtualFrame=Header Frame, Ns_HeaderFrameID=0, Ns_VirtualFrameStatusFlg=off, Ns_IncompleteFrameCntFlg=off, Ns_OverflowCntFlg=off, Ns_FrameBufferSize=1, Ns_SampleTime=0.05}
      | uint16(Ns_DeviceID),
      | uint16(Ns_ChannelNum),
      | uint32(Ns_FrameID),
      | uint8(Ns_IsVirtualFrame),
      | uint16(Ns_RoleInVirtualFrame),
      | uint32(Ns_HeaderFrameID),
      | uint8(Ns_VirtualFrameStatusFlg),
      | uint8(Ns_IncompleteFrameCntFlg),
      | uint8(Ns_OverflowCntFlg),
      | uint16(Ns_FrameBufferSize),
      | double(Ns_SampleTime)
      mask prompts: Ns_DeviceID "Device:"; Ns_ChannelNum "Channel number:"; Ns_FrameID "Frame ID:"; Ns_IsVirtualFrame "Belong to a virtual frame"; Ns_RoleInVirtualFrame "Position in virtual frame:"; Ns_HeaderFrameID "Header frame ID:"; Ns_VirtualFrameStatusFlg "Current virtural frame status output"; Ns_IncompleteFrameCntFlg "Incomplete virtual frame count output"; Ns_OverflowCntFlg "Overflow count output"; Ns_FrameBufferSize "Frame buffer size:"; Ns_SampleTime "Sample time:"
      mask init:
      | NSTC297CANReceive_callback('portlabels');
      mask TypeOptions Ns_DeviceID: General Control Unit Gen2 | ADAS Control Unit Gen2
      mask TypeOptions Ns_ChannelNum: 0 | 1 | 2 | 3 | 4 | 5
      mask Callback Ns_IsVirtualFrame: NSTC297CANReceive_callback('Belong to a virtual frame');
      mask TypeOptions Ns_RoleInVirtualFrame: Header Frame | Data Frame | Trailer Frame
      mask Callback Ns_RoleInVirtualFrame: NSTC297CANReceive_callback('Position in virtual frame');
      mask Display: color('blue');text(0.02,0.9,'NovSteeds TC297','horizontalAlignment','left');color('blue');text(0.5,0.7,'CAN Receive','horizontalAlignment','center');color('black');text(0.5,0.6,'Channel: 5','horizontalAlignment','center');text(0.5,0.5,'ID: 1534','horizontalAlignment','center');text(0.5,0.4,'Virtual Frame: No','horizontalAlignment','center');port_label('output',1, 'RemainderCnt');port_label('output',2, 'Msg');
  Time Limit : Constant  Commented=on  OutDataTypeStr=single  SampleTime=-1
  R0Info_facmR0C0 : Outport
  R0Info_facmR0C1 : Outport  Port=2
  R0Info_facmR0C2 : Outport  Port=3
  R0Info_facmR0C3 : Outport  Port=4
  R0Info_facmR0Ql : Outport  Port=5
  R0Info_efR0FaultSyn : Outport  Port=6
  wires:
  Data Type Conversion4/1 -> R0Info_facmR0C0/1
  Data Type Conversion5/1 -> R0Info_facmR0Ql/1
  Data Type Conversion3/1 -> R0Info_facmR0C3/1
  Data Type Conversion2/1 -> R0Info_facmR0C2/1
  Data Type Conversion1/1 -> R0Info_facmR0C1/1
  CAN Receive (CANRX)/2 -> CAN Unpack14/1, CAN Diagnosis (CANDia)/4(CANDia_regCANMsg)
  CAN Receive (CANRX)/1 -> CAN Diagnosis (CANDia)/3(CANDia_cfNewFlg)
  Time Limit/1 -> CAN Diagnosis (CANDia)/2(CANDia_tiTLim)
  CAN Receive Sample Time/1 -> CAN Diagnosis (CANDia)/1(CANDia_tiCANRxSmplT)
  ? -> CAN Diagnosis (CANDia)/5(CANDia_ctRllCnt)
  R0 Information Fault Synthesis (R0FaultSyn)/1(R0FaultSyn_efL0FaultSyn) -> R0Info_efR0FaultSyn/1
  S-Function3/2 -> CAN Unpack3/1
  CAN Unpack3/1 -> Data Type Conversion4/1
  CAN Unpack3/2 -> Data Type Conversion1/1
  CAN Unpack3/3 -> Data Type Conversion2/1
  CAN Unpack3/4 -> Data Type Conversion3/1
  CAN Unpack3/7 -> Data Type Conversion5/1

== system DFADAS2_SenFus_v1_201204RC_training_210115/Signal Input (Input)/Signal Input (50ms) (Input50)/Front Left Radar(S2) Objects Information (FLRdr)/S0 Data Frame Read/Enabled Subsystem ==
  note: Reset
  RemainderCnt : Inport
  Msg : Inport  Port=2
  obj_num : Inport  Port=3
  Enable : EnablePort  StatesWhenEnabling=reset
  Bus Creator : BusCreator  Inputs=10
  M0ObjInfo : Subsystem  TreatAsAtomicUnit=on
  M1ObjInfo1 : Subsystem  TreatAsAtomicUnit=on
  M2ObjInfo : Subsystem  TreatAsAtomicUnit=on
  M3ObjInfo : Subsystem  TreatAsAtomicUnit=on
  M4ObjInfo1 : Subsystem  TreatAsAtomicUnit=on
  Unpack : Subsystem
  RLRdrObjInfo : Outport
  wires:
  obj_num/1 -> M0ObjInfo/4(obj_num), M1ObjInfo1/4(obj_num), M2ObjInfo/4(obj_num), M3ObjInfo/4(obj_num), M4ObjInfo1/4(obj_num)
  M3ObjInfo/2(M31ObjInfo) -> Bus Creator/8  "M31ObjInfo"
  M4ObjInfo1/2(M41ObjInfo) -> Bus Creator/10  "M41ObjInfo"
  M2ObjInfo/2(M21ObjInfo) -> Bus Creator/6  "M21ObjInfo"
  M1ObjInfo1/2(M11ObjInfo) -> Bus Creator/4  "M11ObjInfo"
  M0ObjInfo/2(M01ObjInfo) -> Bus Creator/2  "M01ObjInfo"
  Unpack/2(MValue) -> M0ObjInfo/2(MValue), M1ObjInfo1/2(MValue), M2ObjInfo/2(MValue), M3ObjInfo/2(MValue), M4ObjInfo1/2(MValue)
  RemainderCnt/1 -> M1ObjInfo1/3(RemainderCnt), M2ObjInfo/3(RemainderCnt), M3ObjInfo/3(RemainderCnt), M4ObjInfo1/3(RemainderCnt), M0ObjInfo/3(RemainderCnt), Unpack/2(RemainderCnt)
  Bus Creator/1 -> RLRdrObjInfo/1  "RLRdrObjInfo"
  M4ObjInfo1/1(M40ObjInfo) -> Bus Creator/9  "M40ObjInfo"
  M3ObjInfo/1(M30ObjInfo) -> Bus Creator/7  "M30ObjInfo"
  M2ObjInfo/1(M20ObjInfo) -> Bus Creator/5  "M20ObjInfo"
  M1ObjInfo1/1(M10ObjInfo) -> Bus Creator/3  "M10ObjInfo"
  M0ObjInfo/1(M00ObjInfo) -> Bus Creator/1  "M00ObjInfo"
  Unpack/1(MsgOut) -> M1ObjInfo1/1(msg), M2ObjInfo/1(msg), M3ObjInfo/1(msg), M4ObjInfo1/1(msg), M0ObjInfo/1(msg)
  Msg/1 -> Unpack/1(Msg)
